simulink model "FORWARDSIM"  (R2021a)
settings: Solver=ode45  StartTime=0.0  StopTime=10.0  RelTol=1e-3  EnableMultiTasking=on
settings Model: Creator=Dell  LastModifiedBy=Islam Barakat
settings SolverCC: AlgebraicLoopSolver=TrustRegion
settings DataIOCC: LimitDataPoints=on  SaveFormat=Array  ReturnWorkspaceOutputs=off
settings OptimizationCC: LifeSpan=inf
settings DebuggingCC: SolverPrmCheckMsg=warning  SFUnexpectedBacktrackingDiag=warning  SFNoUnconditionalDefaultTransitionDiag=warning  SFExecutionAtInitializationDiag=none  SFMachineParentedDataDiag=warning  ArithmeticOperatorsInVariantConditions=warning
settings HardwareCC: ProdBitPerPointer=32  ProdBitPerSizeT=32  ProdBitPerPtrDiffT=32  ProdLargestAtomicFloat=None  ProdIntDivRoundTo=Undefined  ProdEndianess=Unspecified  ProdWordSize=32  ProdHWDeviceType=32-bit Generic
settings ModelReferenceCC: PropagateSignalLabelsOutOfModel=off
settings SFSimCC: SimUseLocalCustomCode=off  CustomCodeUndefinedFunction=UseInterfaceOnly
settings RTWCC: RTWUseLocalCustomCode=off
settings CodeAppCC: StateflowObjectComments=on
settings GRTTargetCC: TargetLangStandard=C89/C90 (ANSI)
settings ConfigComp: CovMetricSettings=dw  CovSaveCumulativeToWorkspaceVar=on  CovSaveSingleToWorkspaceVar=on  CovExternalEMLEnable=off  CovSFcnEnable=off

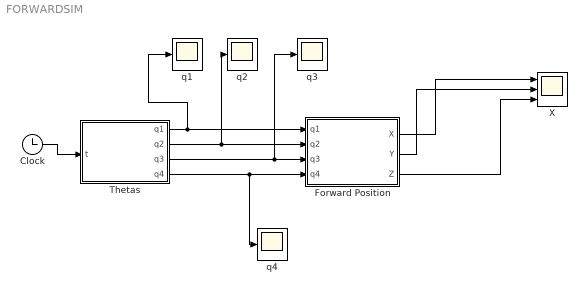
== system FORWARDSIM ==
  Clock : Clock
  Forward Position : MATLAB Function  TreatAsAtomicUnit=on
  Thetas : MATLAB Function  TreatAsAtomicUnit=on
  X : Scope  NumInputPorts=3
  q{1..4} (4 alike) : Scope
  wires:
  Clock/1 -> Thetas/1(t)
  Thetas/1(q1) -> q1/1, Forward Position/1(q1)
  Thetas/2(q2) -> q2/1, Forward Position/2(q2)
  Thetas/3(q3) -> q3/1, Forward Position/3(q3)
  Thetas/4(q4) -> q4/1, Forward Position/4(q4)
  Forward Position/1(X) -> X/1
  Forward Position/2(Y) -> X/2
  Forward Position/3(Z) -> X/3

== matlab function FORWARDSIM/Forward Position ==
  data: q1 input; X output; q2 input; q3 input; q4 input; Y output; Z output
function [X,Y,Z] = fcn(q1,q2,q3,q4)
 
X=  120*cos(q4)*(sin(q1)*sin(q3) + cos(q1)*cos(q2)*cos(q3)) - (537*cos(q1)*sin(q2))/5 - 120*cos(q1)*sin(q2)*sin(q4);
Y= - (537*sin(q1)*sin(q2))/5 - 120*cos(q4)*(cos(q1)*sin(q3) - cos(q2)*cos(q3)*sin(q1)) - 120*sin(q1)*sin(q2)*sin(q4);
Z= 81/2 - 120*cos(q2)*sin(q4) - 120*cos(q3)*cos(q4)*sin(q2) - (537*cos(q2))/5;


end

== matlab function FORWARDSIM/Thetas ==
  data: t input; q1 output; q2 output; q3 output; q4 output
function [q1,q2,q3,q4] = fcn(t)
%#codegen
q1=pi/2;
q2=pi/2;
q3=pi/2;
q4=pi/2;

end
